simulink model "CPM_f0"  (R2023a)
settings: Solver=VariableStepAuto  StartTime=0.0  StopTime=6  RelTol=1e-3
values from neighbouring files (symbols this model uses):
  A = sqrt(2*E/sampleTime)    [dataCPM.m]
  f_0 = 2000000    [dataCPM.m]
  f_1 = f_0 + f    (= 2000000.25)    [dataCPM.m]
  f_2 = f_0 - f    (= 1999999.75)    [dataCPM.m]
  sampleTime = 1    [dataCPM.m]
libraries: simulink_extras x4, commdigbbndcpm2 x2
settings Model: Creator=mluser  LastModifiedBy=x
settings DebuggingCC: ParameterOverflowMsg=none  ParameterUnderflowMsg=error

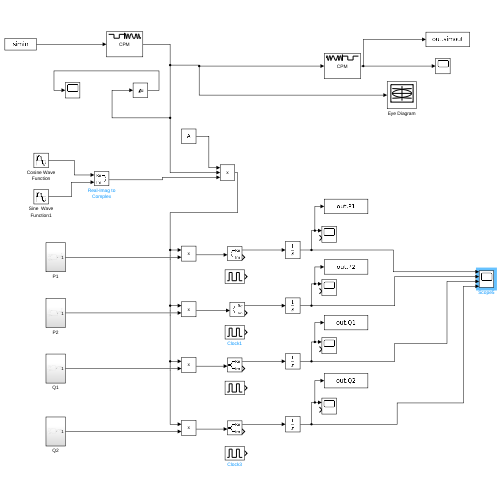
[thumbnail: Simulink's stored preview of the top-level diagram]
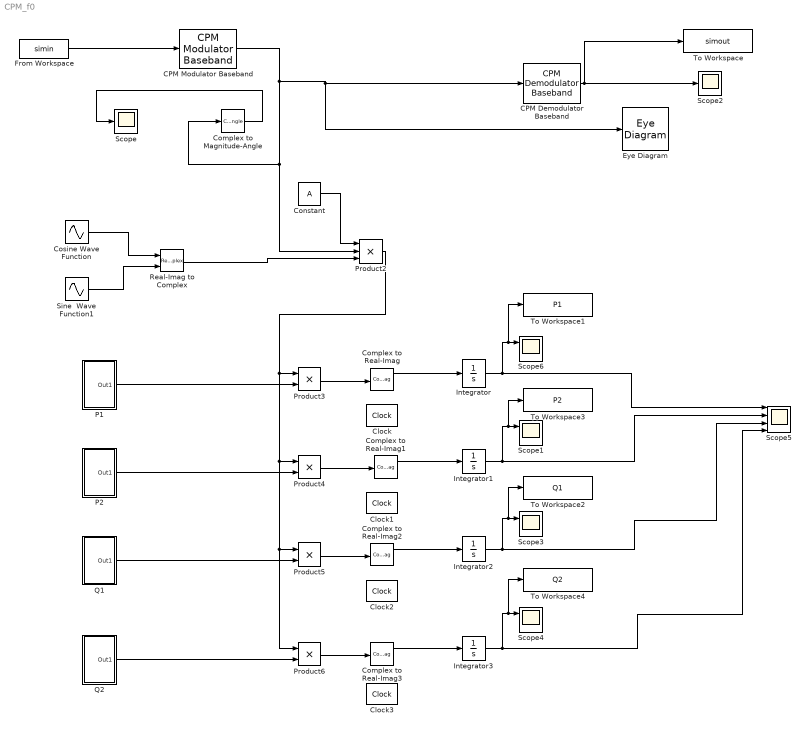
== system CPM_f0 ==
  CPM Demodulator Baseband : commdigbbndcpm2/CPM Demodulator Baseband  Mnum=2  outputType=Integer  mappingType=Binary  modIdx=0.5  pulseShape=Rectangular  BT=0.3  mainLobePulseLength=1  rollOff=0.2  pulseLength=1  preHistory=1  phaseOffset=0  samplesPerSymbol=32  RateOptions=Allow multirate processing  traceBack=1  outDType=double
  CPM Modulator Baseband : commdigbbndcpm2/CPM Modulator Baseband  Mnum=2  inputType=Integer  mappingType=Binary  modIdx=0.5  pulseShape=Rectangular  BT=0.3  mainLobePulseLength=1  rollOff=0.2  pulseLength=1  preHistory=1  phaseOffset=0  samplesPerSymbol=32  RateOptions=Allow multirate processing  outDataType=double
  Clock{,1..3} (4 alike) : simulink_extras/Flip Flops/Clock  period=1
  Complex to Magnitude-Angle : ComplexToMagnitudeAngle  Output=Angle
  Complex to Real-Imag{,1..3} (4 alike) : ComplexToRealImag
  Constant : Constant  Value=A
  Cosine Wave Function : Sin  Amplitude=A  Frequency=f_0  Phase=pi/2  SampleTime=1/32
  Eye Diagram : EyeDiagram
  From Workspace : FromWorkspace  VariableName=simin  OutDataTypeStr=double  SampleTime=sampleTime  Interpolate=off  OutputAfterFinalValue=Holding final value
  Integrator{,1..3} (4 alike) : Integrator
  P1 : Subsystem
  P2 : Subsystem
  Product2 : Product  Inputs=3
  Product{3..6} (4 alike) : Product
  Q1 : Subsystem
  Q2 : Subsystem
  Real-Imag to Complex : RealImagToComplex
  Scope : Scope
  Scope{1,3..4,6} (4 alike) : Scope  NumInputPorts=2
  Scope2 : Scope
  Scope5 : Scope  NumInputPorts=4
  Sine  Wave Function1 : Sin  Amplitude=A  Frequency=f_0  SampleTime=1/32
  To Workspace : ToWorkspace  VariableName=simout  SampleTime=-1
      settings: Save2DSignal=2-D array (concatenate along first dimension)
  To Workspace1 : ToWorkspace  VariableName=P1  SampleTime=1
      settings: Save2DSignal=2-D array (concatenate along first dimension)
  To Workspace2 : ToWorkspace  VariableName=Q1  SampleTime=1
      settings: Save2DSignal=2-D array (concatenate along first dimension)
  To Workspace3 : ToWorkspace  VariableName=P2  SampleTime=1
      settings: Save2DSignal=2-D array (concatenate along first dimension)
  To Workspace4 : ToWorkspace  VariableName=Q2  SampleTime=1
      settings: Save2DSignal=2-D array (concatenate along first dimension)
  wires:
  From Workspace/1 -> CPM Modulator Baseband/1
  CPM Demodulator Baseband/1 -> To Workspace/1, Scope2/1
  CPM Modulator Baseband/1 -> Product2/2, Complex to Magnitude-Angle/1, Eye Diagram/1, CPM Demodulator Baseband/1
  Complex to Magnitude-Angle/1 -> Scope/1
  Constant/1 -> Product2/1
  Product2/1 -> Product6/1, Product5/1, Product4/1, Product3/1
  Q2/1(Out1) -> Product6/2
  Q1/1(Out1) -> Product5/2
  P2/1(Out1) -> Product4/2
  P1/1(Out1) -> Product3/2
  Integrator/1 -> Scope5/1, To Workspace1/1, Scope6/1
  Product3/1 -> Complex to Real-Imag/1
  Complex to Real-Imag/1 -> Integrator/1
  Product4/1 -> Complex to Real-Imag1/1
  Complex to Real-Imag1/1 -> Integrator1/1
  Integrator1/1 -> Scope5/2, To Workspace3/1, Scope1/1
  Product5/1 -> Complex to Real-Imag2/1
  Complex to Real-Imag2/1 -> Integrator2/1
  Integrator2/1 -> Scope5/3, To Workspace2/1, Scope3/1
  Product6/1 -> Complex to Real-Imag3/1
  Complex to Real-Imag3/1 -> Integrator3/1
  Integrator3/1 -> Scope5/4, To Workspace4/1, Scope4/1
  Cosine Wave Function/1 -> Real-Imag to Complex/1
  Sine  Wave Function1/1 -> Real-Imag to Complex/2
  Real-Imag to Complex/1 -> Product2/3

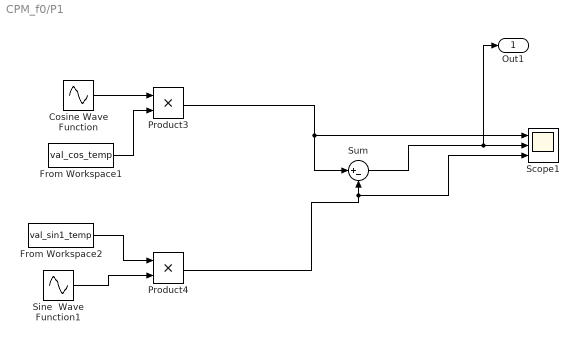
== system CPM_f0/P1 ==
  Cosine Wave Function : Sin  Amplitude=A  Frequency=f_1  Phase=pi/2  SampleTime=1/32
  From Workspace1 : FromWorkspace  VariableName=val_cos_temp  SampleTime=sampleTime  OutputAfterFinalValue=Holding final value
  From Workspace2 : FromWorkspace  VariableName=val_sin1_temp  SampleTime=sampleTime  OutputAfterFinalValue=Holding final value
  Product3 : Product
  Product4 : Product
  Scope1 : Scope  NumInputPorts=3
  Sine  Wave Function1 : Sin  Amplitude=A  Frequency=f_1  SampleTime=1/32
  Sum : Sum  Inputs=|+-
  Out1 : Outport
  wires:
  Sum/1 -> Out1/1, Scope1/2
  From Workspace1/1 -> Product3/2
  Cosine Wave Function/1 -> Product3/1
  Sine  Wave Function1/1 -> Product4/2
  Product4/1 -> Scope1/3, Sum/2
  Product3/1 -> Sum/1, Scope1/1
  From Workspace2/1 -> Product4/1

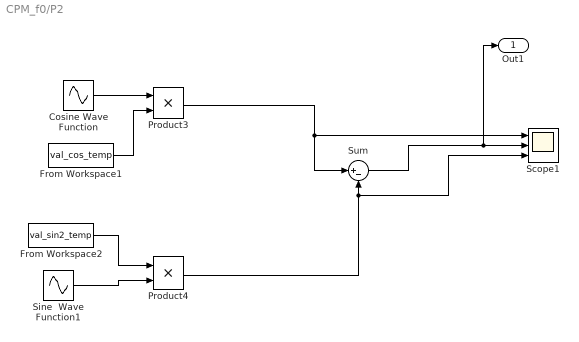
== system CPM_f0/P2 ==
  Cosine Wave Function : Sin  Amplitude=A  Frequency=f_2  Phase=pi/2  SampleTime=1/32
  From Workspace1 : FromWorkspace  VariableName=val_cos_temp  SampleTime=sampleTime  OutputAfterFinalValue=Holding final value
  From Workspace2 : FromWorkspace  VariableName=val_sin2_temp  SampleTime=sampleTime  OutputAfterFinalValue=Holding final value
  Product3 : Product
  Product4 : Product
  Scope1 : Scope  NumInputPorts=3
  Sine  Wave Function1 : Sin  Amplitude=A  Frequency=f_2  SampleTime=1/32
  Sum : Sum  Inputs=|+-
  Out1 : Outport
  wires:
  Sum/1 -> Out1/1, Scope1/2
  From Workspace1/1 -> Product3/2
  Cosine Wave Function/1 -> Product3/1
  Sine  Wave Function1/1 -> Product4/2
  Product4/1 -> Scope1/3, Sum/2
  Product3/1 -> Sum/1, Scope1/1
  From Workspace2/1 -> Product4/1

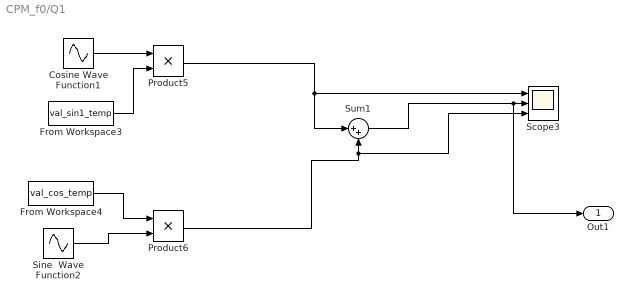
== system CPM_f0/Q1 ==
  Cosine Wave Function1 : Sin  Amplitude=A  Frequency=f_1  Phase=pi/2  SampleTime=1/32
  From Workspace3 : FromWorkspace  VariableName=val_sin1_temp  SampleTime=sampleTime  OutputAfterFinalValue=Holding final value
  From Workspace4 : FromWorkspace  VariableName=val_cos_temp  SampleTime=sampleTime  OutputAfterFinalValue=Holding final value
  Product5 : Product
  Product6 : Product
  Scope3 : Scope  NumInputPorts=3
  Sine  Wave Function2 : Sin  Amplitude=A  Frequency=f_1  SampleTime=1/32
  Sum1 : Sum  Inputs=|++
  Out1 : Outport
  wires:
  From Workspace3/1 -> Product5/2
  Sine  Wave Function2/1 -> Product6/2
  Cosine Wave Function1/1 -> Product5/1
  From Workspace4/1 -> Product6/1
  Product6/1 -> Scope3/3, Sum1/2
  Sum1/1 -> Out1/1, Scope3/2
  Product5/1 -> Sum1/1, Scope3/1

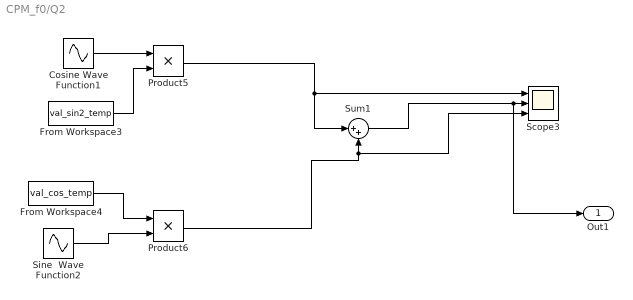
== system CPM_f0/Q2 ==
  Cosine Wave Function1 : Sin  Amplitude=A  Frequency=f_2  Phase=pi/2  SampleTime=1/32
  From Workspace3 : FromWorkspace  VariableName=val_sin2_temp  SampleTime=sampleTime  OutputAfterFinalValue=Holding final value
  From Workspace4 : FromWorkspace  VariableName=val_cos_temp  SampleTime=sampleTime  OutputAfterFinalValue=Holding final value
  Product5 : Product
  Product6 : Product
  Scope3 : Scope  NumInputPorts=3
  Sine  Wave Function2 : Sin  Amplitude=A  Frequency=f_2  SampleTime=1/32
  Sum1 : Sum  Inputs=|++
  Out1 : Outport
  wires:
  From Workspace3/1 -> Product5/2
  Sine  Wave Function2/1 -> Product6/2
  Cosine Wave Function1/1 -> Product5/1
  From Workspace4/1 -> Product6/1
  Product6/1 -> Scope3/3, Sum1/2
  Sum1/1 -> Out1/1, Scope3/2
  Product5/1 -> Sum1/1, Scope3/1
